simulink subsystem "rss_load_model"  (R2023a)
settings: Solver=VariableStepAuto  StartTime=0.0  StopTime=10.0  RelTol=1e-3
settings Model: Creator=cav2ofo  LastModifiedBy=lenovo
settings OptimizationCC: ReuseModelBlockBuffer=off

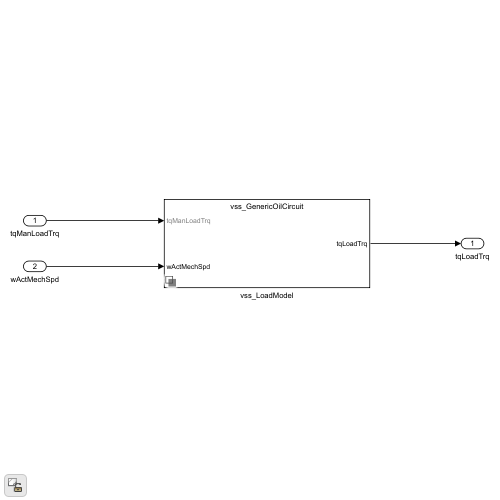
[thumbnail: Simulink's stored preview of the top-level diagram]
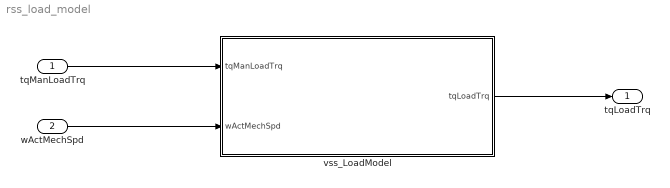
== system rss_load_model ==
  tqManLoadTrq : Inport
  wActMechSpd : Inport  Port=2
  vss_LoadModel : Subsystem  Variant=on  VariantControlMode=label  LabelModeActiveChoice=parCompMdlVrs1
  tqLoadTrq : Outport
  wires:
  tqManLoadTrq/1 -> vss_LoadModel/1(tqManLoadTrq)
  wActMechSpd/1 -> vss_LoadModel/2(wActMechSpd)
  vss_LoadModel/1(tqLoadTrq) -> tqLoadTrq/1

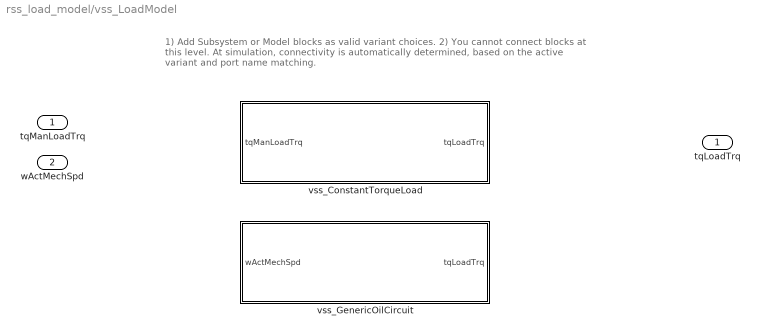
== system rss_load_model/vss_LoadModel ==
  note: 1) Add Subsystem or Model blocks as valid variant choices.
      | 2) You cannot connect blocks at this level. At simulation, connectivity is automatically
      | determined, based on the active variant and port name matching.
  tqManLoadTrq : Inport
  wActMechSpd : Inport  Port=2
  vss_ConstantTorqueLoad : Subsystem  VariantControl=parSmplMdl
  vss_GenericOilCircuit : Subsystem  VariantControl=parCompMdlVrs1
  tqLoadTrq : Outport

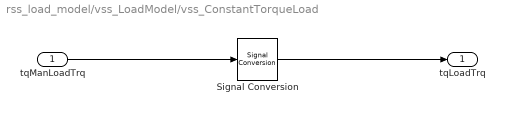
== system rss_load_model/vss_LoadModel/vss_ConstantTorqueLoad ==
  tqManLoadTrq : Inport
  Signal Conversion : SignalConversion  OverrideOpt=off
  tqLoadTrq : Outport
  wires:
  Signal Conversion/1 -> tqLoadTrq/1
  tqManLoadTrq/1 -> Signal Conversion/1

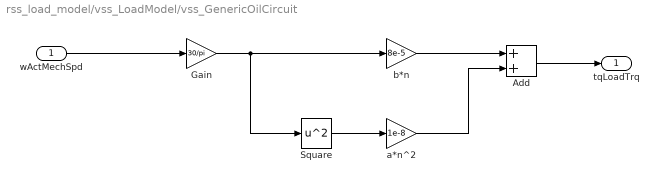
== system rss_load_model/vss_LoadModel/vss_GenericOilCircuit ==
  wActMechSpd : Inport
  Add : Sum
  Gain : Gain  Gain=30/pi
  Square : Math  Operator=square
  a*n^2 : Gain  Gain=1e-8
  b*n : Gain  Gain=8e-5
  tqLoadTrq : Outport
  wires:
  a*n^2/1 -> Add/2
  b*n/1 -> Add/1
  Square/1 -> a*n^2/1
  Gain/1 -> b*n/1, Square/1
  Add/1 -> tqLoadTrq/1
  wActMechSpd/1 -> Gain/1
